simulink model "two_DOF_Translational_system"  (R2024b)
settings: Solver=VariableStepAuto  StartTime=0.0  StopTime=Sim_Time  RelTol=1e-3
undefined symbols (not defined in the file): F, fv1, fv2, fv3, k1, k2, k3, M1, M2
settings Model: Creator=Lenovo  LastModifiedBy=Lenovo

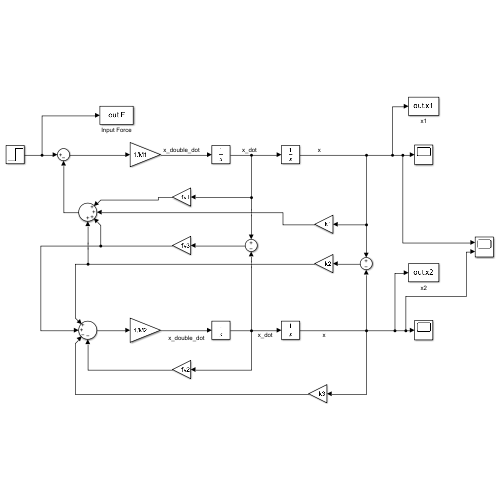
[thumbnail: Simulink's stored preview of the top-level diagram]
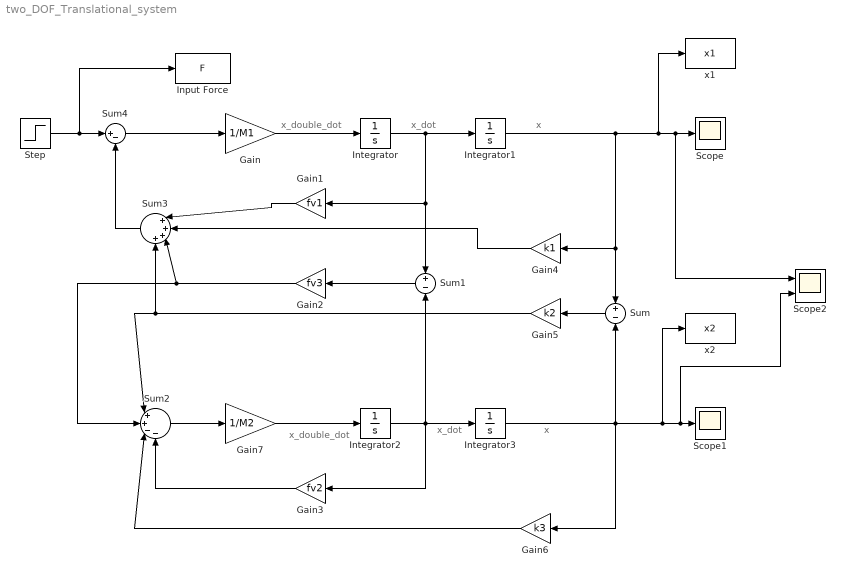
== system two_DOF_Translational_system ==
  note: x_double_dot
  note: x_dot
  note: x
  note: x_double_dot
  note: x_dot
  note: x
  Gain : Gain  Gain=1/M1
  Gain1 : Gain  Gain=fv1
  Gain2 : Gain  Gain=fv3
  Gain3 : Gain  Gain=fv2
  Gain4 : Gain  Gain=k1
  Gain5 : Gain  Gain=k2
  Gain6 : Gain  Gain=k3
  Gain7 : Gain  Gain=1/M2
  Input Force : ToWorkspace  VariableName=F  SaveFormat=Timeseries  SampleTime=-1
  Integrator{,1..3} (4 alike) : Integrator
  Scope : Scope
  Scope1 : Scope
  Scope2 : Scope  NumInputPorts=2
  Step : Step  After=F  SampleTime=0
  Sum : Sum  Inputs=+-
  Sum1 : Sum  Inputs=+-
  Sum2 : Sum  Inputs=|++--
  Sum3 : Sum  Inputs=|++++
  Sum4 : Sum  Inputs=|+-
  x1 : ToWorkspace  VariableName=x1  SaveFormat=Timeseries  SampleTime=-1
  x2 : ToWorkspace  VariableName=x2  SaveFormat=Timeseries  SampleTime=-1
  wires:
  Integrator/1 -> Sum1/1, Gain1/1, Integrator1/1
  Gain/1 -> Integrator/1
  Integrator1/1 -> x1/1, Scope2/1, Scope/1, Gain4/1, Sum/1
  Gain7/1 -> Integrator2/1
  Integrator2/1 -> Gain3/1, Sum1/2, Integrator3/1
  Integrator3/1 -> x2/1, Scope2/2, Scope1/1, Gain6/1, Sum/2
  Sum/1 -> Gain5/1
  Sum1/1 -> Gain2/1
  Sum2/1 -> Gain7/1
  Gain3/1 -> Sum2/4
  Gain6/1 -> Sum2/3
  Gain5/1 -> Sum3/4, Sum2/1
  Gain2/1 -> Sum3/3, Sum2/2
  Gain4/1 -> Sum3/2
  Gain1/1 -> Sum3/1
  Sum3/1 -> Sum4/2
  Step/1 -> Input Force/1, Sum4/1
  Sum4/1 -> Gain/1
